simulink model "joystickcalibtest"  (Simulink 9.1)
settings: Solver=ode45  StartTime=0.0  StopTime=Inf  RelTol=1e-3  EnableMultiTasking=on
libraries: vrlib x1
settings Model: Creator=tjjlombaerts  LastModifiedBy=jelle
settings DataIOCC: LimitDataPoints=on  SignalLoggingSaveFormat=ModelDataLogs  SignalLoggingName=sigsOut
settings OptimizationCC: ExpressionDepthLimit=2147483647  InitFltsAndDblsToZero=on
settings DebuggingCC: SaveWithParameterizedLinksMsg=none  SignalResolutionControl=TryResolveAllWithWarning  MultiTaskDSMMsg=warning  MultiTaskCondExecSysMsg=none  FcnCallInpInsideContextMsg=warning  StateNameClashWarn=warning
settings HardwareCC: TargetUnknown=on

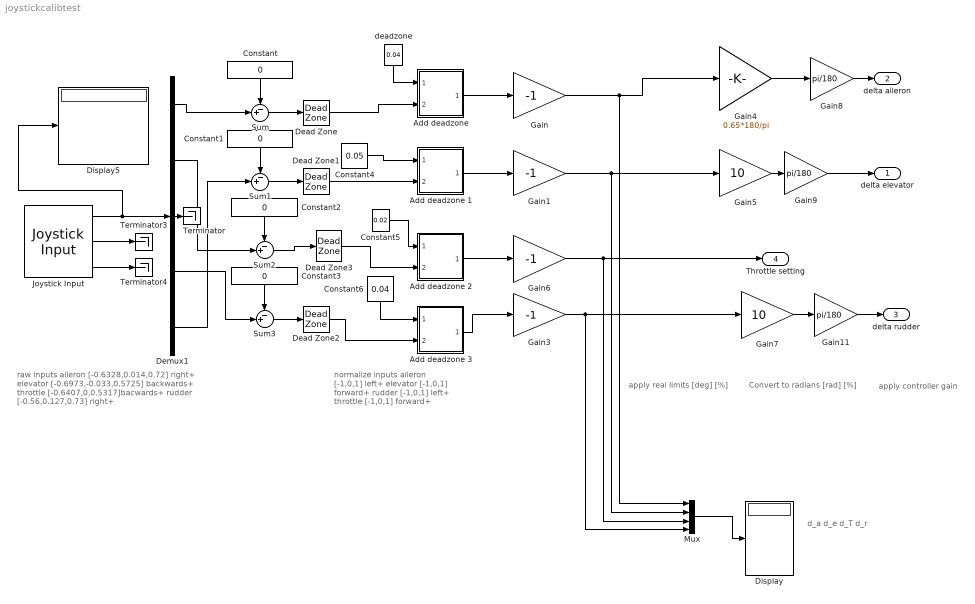
== system joystickcalibtest ==
  note: d_a
      | d_e
      | d_T
      | d_r
  note: raw inputs
      | aileron [-0.6328,0.014,0.72] right+
      | elevator [-0.6973,-0.033,0.5725] backwards+
      | throttle [-0.6407,0,0.5317]bacwards+
      | rudder [-0.56,0.127,0.73] right+
  note: normalize inputs
      | aileron [-1,0,1] left+
      | elevator [-1,0,1] forward+
      | rudder [-1,0,1] left+
      | throttle [-1,0,1] forward+
  note: apply real limits
      | [deg]
      | [%]
  note: Convert to radians
      | [rad]
      | [%]
  note: apply controller
      | gain
  " deadzone " : Constant  Value=0.04
  "Add deadzone " : Subsystem
  Add deadzone 1 : Subsystem
  Add deadzone 2 : Subsystem
  Add deadzone 3 : Subsystem
  Constant{,1..3} (4 alike) : Constant  Value=0
  Constant4 : Constant  Value=0.05
  Constant5 : Constant  Value=0.02
  Constant6 : Constant  Value=0.04
  Dead Zone : DeadZone  LowerValue=-0.04  UpperValue=0.04  SaturateOnIntegerOverflow=on
  Dead Zone1 : DeadZone  LowerValue=-0.05  UpperValue=0.05  SaturateOnIntegerOverflow=on
  Dead Zone2 : DeadZone  LowerValue=-0.04  UpperValue=0.04  SaturateOnIntegerOverflow=on
  Dead Zone3 : DeadZone  LowerValue=-0.02  UpperValue=0.02  SaturateOnIntegerOverflow=on
  Demux1 : Demux  Outputs=5
  Display : Display
  Display5 : Display
  Gain{,1,3,6} (4 alike) : Gain  Gain=-1  SaturateOnIntegerOverflow=on  OutDataTypeStr=Inherit: Same as input  ParamDataTypeStr=Inherit: Same as input
  Gain11 : Gain  Gain=pi/180  SaturateOnIntegerOverflow=on  OutDataTypeStr=Inherit: Same as input  ParamDataTypeStr=Inherit: Same as input
  Gain4 : Gain  Gain=0.65*180/pi  SaturateOnIntegerOverflow=on  OutDataTypeStr=Inherit: Same as input  ParamDataTypeStr=Inherit: Same as input
  Gain5 : Gain  Gain=10  SaturateOnIntegerOverflow=on  OutDataTypeStr=Inherit: Same as input  ParamDataTypeStr=Inherit: Same as input
  Gain7 : Gain  Gain=10  SaturateOnIntegerOverflow=on  OutDataTypeStr=Inherit: Same as input  ParamDataTypeStr=Inherit: Same as input
  Gain8 : Gain  Gain=pi/180  SaturateOnIntegerOverflow=on  OutDataTypeStr=Inherit: Same as input  ParamDataTypeStr=Inherit: Same as input
  Gain9 : Gain  Gain=pi/180  SaturateOnIntegerOverflow=on  OutDataTypeStr=Inherit: Same as input  ParamDataTypeStr=Inherit: Same as input
  Joystick Input : vrlib/Joystick Input  joyid=1  adjustports=on  forcefeed=off
      settings: SourceProductBaseCode=VR
  Mux : Mux
  Sum{,1..3} (4 alike) : Sum  Inputs=-+|  SaturateOnIntegerOverflow=on
  Terminator : Terminator
  Terminator3 : Terminator
  Terminator4 : Terminator
  delta elevator : Outport
  delta aileron : Outport  Port=2
  delta rudder : Outport  Port=3
  Throttle setting : Outport  Port=4
  wires:
  Joystick Input/1 -> Display5/1, Demux1/1
  Joystick Input/2 -> Terminator3/1
  Joystick Input/3 -> Terminator4/1
  Demux1/1 -> Sum/2
  Constant/1 -> Sum/1
  Constant1/1 -> Sum1/1
  Constant2/1 -> Sum2/1
  Constant3/1 -> Sum3/1
  Sum/1 -> Dead Zone/1
  Gain/1 -> Mux/1, Gain4/1
  Sum1/1 -> Dead Zone1/1
  Gain1/1 -> Gain5/1, Mux/2
  Sum2/1 -> Dead Zone3/1
  Sum3/1 -> Dead Zone2/1
  Gain3/1 -> Mux/4, Gain7/1
  Gain4/1 -> Gain8/1
  Gain5/1 -> Gain9/1
  Gain6/1 -> Mux/3, Throttle setting/1
  Gain7/1 -> Gain11/1
  Gain8/1 -> delta aileron/1
  Gain9/1 -> delta elevator/1
  Gain11/1 -> delta rudder/1
  Demux1/4 -> Sum3/2
  Demux1/2 -> Sum2/2
  Demux1/5 -> Sum1/2
  "Add deadzone "/1(Out1) -> Gain/1
  " deadzone "/1 -> "Add deadzone "/1("Value  ")
  Dead Zone/1 -> "Add deadzone "/2("Input ")
  Dead Zone1/1 -> Add deadzone 1/2("Input ")
  Constant4/1 -> Add deadzone 1/1("Value  ")
  Add deadzone 1/1(Out1) -> Gain1/1
  Dead Zone3/1 -> Add deadzone 2/2("Input ")
  Constant5/1 -> Add deadzone 2/1("Value  ")
  Add deadzone 2/1(Out1) -> Gain6/1
  Constant6/1 -> Add deadzone 3/1("Value  ")
  Dead Zone2/1 -> Add deadzone 3/2("Input ")
  Add deadzone 3/1(Out1) -> Gain3/1
  Mux/1 -> Display/1
  Demux1/3 -> Terminator/1

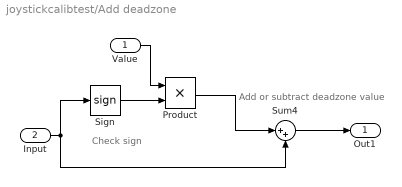
== system joystickcalibtest/Add deadzone  ==
  note: Add or subtract deadzone value
  note: Check sign
  "Value  " : Inport
  "Input " : Inport  Port=2
  Product : Product
  Sign : Signum
  Sum4 : Sum  Inputs=|++
  Out1 : Outport
  wires:
  "Input "/1 -> Sign/1, Sum4/2
  Product/1 -> Sum4/1
  "Value  "/1 -> Product/1
  Sum4/1 -> Out1/1
  Sign/1 -> Product/2

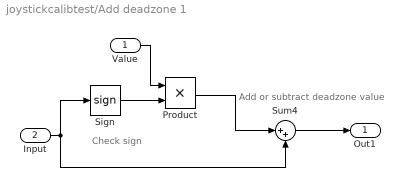
== system joystickcalibtest/Add deadzone 1 ==
  note: Add or subtract deadzone value
  note: Check sign
  "Value  " : Inport
  "Input " : Inport  Port=2
  Product : Product
  Sign : Signum
  Sum4 : Sum  Inputs=|++
  Out1 : Outport
  wires:
  "Input "/1 -> Sign/1, Sum4/2
  Product/1 -> Sum4/1
  "Value  "/1 -> Product/1
  Sum4/1 -> Out1/1
  Sign/1 -> Product/2

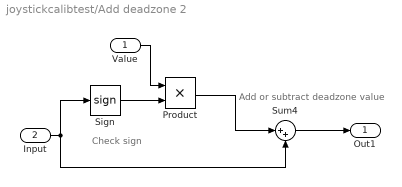
== system joystickcalibtest/Add deadzone 2 ==
  note: Add or subtract deadzone value
  note: Check sign
  "Value  " : Inport
  "Input " : Inport  Port=2
  Product : Product
  Sign : Signum
  Sum4 : Sum  Inputs=|++
  Out1 : Outport
  wires:
  "Input "/1 -> Sign/1, Sum4/2
  Product/1 -> Sum4/1
  "Value  "/1 -> Product/1
  Sum4/1 -> Out1/1
  Sign/1 -> Product/2

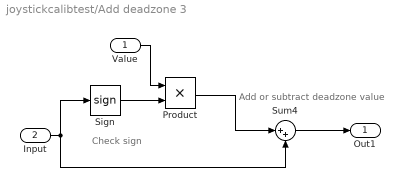
== system joystickcalibtest/Add deadzone 3 ==
  note: Add or subtract deadzone value
  note: Check sign
  "Value  " : Inport
  "Input " : Inport  Port=2
  Product : Product
  Sign : Signum
  Sum4 : Sum  Inputs=|++
  Out1 : Outport
  wires:
  "Input "/1 -> Sign/1, Sum4/2
  Product/1 -> Sum4/1
  "Value  "/1 -> Product/1
  Sum4/1 -> Out1/1
  Sign/1 -> Product/2
